simulink library "halout"  (R2021b)
settings: Solver=VariableStepAuto  StartTime=0.0  StopTime=10.0  RelTol=1e-3
undefined symbols (not defined in the file): C_TASK_5MS_S, FALSE, KHAL_CAN1FD1APS3E2E_flg, KHAL_CAN1FD1APS3TxReq_flg, KHAL_CAN1FD1VCU2E2E_flg, KHAL_CAN1FD1VCU2TxReq_flg, KHAL_CAN1FD1VCU3E2E_flg, KHAL_CAN1FD1VCU3TxReq_flg, KHAL_CAN1TxReq_flg, KHAL_CAN1VMCFCM1E2E_flg, KHAL_CAN1VMCFCM1TxReq_flg, KHAL_CAN2TxReq_flg, KHAL_CAN3FD3VCU1toNIDECTxReq_flg, KHAL_CAN3FD3VCU1TxReq_flg, KHAL_CAN3FD3VCU2E2E_flg, KHAL_CAN3FD3VCU2toNIDECE2E_flg, KHAL_CAN3FD3VCU2toNIDECTxReq_flg, KHAL_CAN3FD3VCU2TxReq_flg, KHAL_CAN3TxReq_flg, KHAL_CAN4FD4CE1000E2E_flg, KHAL_CAN4FD4CE1000TxReq_flg, KHAL_CAN4TxReq_flg, KHAL_CAN5TxReq_flg, KHAL_CAN6FD6APS3E2E_flg, KHAL_CAN6FD6APS3TxReq_flg, KHAL_CAN6FD6VCU2E2E_flg, KHAL_CAN6FD6VCU2TxReq_flg, KHAL_CAN6TxReq_flg, ONE_INT, TRUE, ZERO_INT
libraries: FVT_lib x500, simulink x235
(part 20 of 25)

== system halout/HAL_OUT/CAN3/FD3_VCU2_0x153/Byte_12 ==
  Fr_UdcMax : Inport
  Fr_UdcMin : Inport  Port=2
  BitwiseOR : simulink/Logic and Bit Operations/Bitwise Operator  logicop=OR  UseBitMask=off  NumInputPorts=2  BitMask=bin2dec('11011001')  BitMaskRealWorld=Stored Integer
  SignalPack : FVT_lib/hal/SignalPack  RightShiftCnt=0  BitMask=2^4-1  LeftShiftCnt=4
  SignalPack1 : FVT_lib/hal/SignalPack  RightShiftCnt=8  BitMask=2^4-1  LeftShiftCnt=0
  UnitConverter : DataTypeConversion  OutDataTypeStr=uint8  RndMeth=Round
  UnitConverter1 : DataTypeConversion  OutDataTypeStr=uint16  RndMeth=Round
  UnitConverter2 : DataTypeConversion  OutDataTypeStr=uint8  RndMeth=Round
  UnitConverter3 : DataTypeConversion  OutDataTypeStr=uint16  RndMeth=Round
  Byte_12 : Outport
  wires:
  BitwiseOR/1 -> Byte_12/1
  UnitConverter/1 -> BitwiseOR/1
  SignalPack/1 -> UnitConverter/1
  UnitConverter1/1 -> SignalPack/1
  Fr_UdcMax/1 -> UnitConverter1/1
  UnitConverter2/1 -> BitwiseOR/2
  SignalPack1/1 -> UnitConverter2/1
  UnitConverter3/1 -> SignalPack1/1
  Fr_UdcMin/1 -> UnitConverter3/1

== system halout/HAL_OUT/CAN3/FD3_VCU2_0x153/Byte_13 ==
  Fr_UdcMin : Inport
  BitwiseOR : simulink/Logic and Bit Operations/Bitwise Operator  logicop=OR  UseBitMask=off  BitMask=bin2dec('11011001')  BitMaskRealWorld=Stored Integer
  SignalPack : FVT_lib/hal/SignalPack  RightShiftCnt=0  BitMask=2^8-1  LeftShiftCnt=0
  UnitConverter : DataTypeConversion  OutDataTypeStr=uint8  RndMeth=Round
  UnitConverter1 : DataTypeConversion  OutDataTypeStr=uint16  RndMeth=Round
  Byte_13 : Outport
  wires:
  BitwiseOR/1 -> Byte_13/1
  UnitConverter/1 -> BitwiseOR/1
  SignalPack/1 -> UnitConverter/1
  UnitConverter1/1 -> SignalPack/1
  Fr_UdcMin/1 -> UnitConverter1/1

== system halout/HAL_OUT/CAN3/FD3_VCU2_0x153/Byte_14 ==
  Rr_TMTqReq : Inport
  BitwiseOR : simulink/Logic and Bit Operations/Bitwise Operator  logicop=OR  UseBitMask=off  BitMask=bin2dec('11011001')  BitMaskRealWorld=Stored Integer
  SignalPack : FVT_lib/hal/SignalPack  RightShiftCnt=8  BitMask=2^8-1  LeftShiftCnt=0
  UnitConverter : DataTypeConversion  OutDataTypeStr=uint8  RndMeth=Round
  UnitConverter1 : DataTypeConversion  OutDataTypeStr=uint16  RndMeth=Round
  convert_out : FVT_lib/hal/convert_out  gain=1  offset=-530
  Byte_14 : Outport
  wires:
  BitwiseOR/1 -> Byte_14/1
  UnitConverter/1 -> BitwiseOR/1
  SignalPack/1 -> UnitConverter/1
  UnitConverter1/1 -> SignalPack/1
  convert_out/1 -> UnitConverter1/1
  Rr_TMTqReq/1 -> convert_out/1

== system halout/HAL_OUT/CAN3/FD3_VCU2_0x153/Byte_15 ==
  Rr_TMTqReq : Inport
  BitwiseOR : simulink/Logic and Bit Operations/Bitwise Operator  logicop=OR  UseBitMask=off  BitMask=bin2dec('11011001')  BitMaskRealWorld=Stored Integer
  SignalPack : FVT_lib/hal/SignalPack  RightShiftCnt=0  BitMask=2^8-1  LeftShiftCnt=0
  UnitConverter : DataTypeConversion  OutDataTypeStr=uint8  RndMeth=Round
  UnitConverter1 : DataTypeConversion  OutDataTypeStr=uint16  RndMeth=Round
  convert_out : FVT_lib/hal/convert_out  gain=1  offset=-530
  Byte_15 : Outport
  wires:
  BitwiseOR/1 -> Byte_15/1
  UnitConverter/1 -> BitwiseOR/1
  SignalPack/1 -> UnitConverter/1
  UnitConverter1/1 -> SignalPack/1
  convert_out/1 -> UnitConverter1/1
  Rr_TMTqReq/1 -> convert_out/1

== system halout/HAL_OUT/CAN3/FD3_VCU2_0x153/Byte_16 ==
  Fr_TMTqReq : Inport
  BitwiseOR : simulink/Logic and Bit Operations/Bitwise Operator  logicop=OR  UseBitMask=off  BitMask=bin2dec('11011001')  BitMaskRealWorld=Stored Integer
  SignalPack : FVT_lib/hal/SignalPack  RightShiftCnt=8  BitMask=2^8-1  LeftShiftCnt=0
  UnitConverter : DataTypeConversion  OutDataTypeStr=uint8  RndMeth=Round
  UnitConverter1 : DataTypeConversion  OutDataTypeStr=uint16  RndMeth=Round
  convert_out : FVT_lib/hal/convert_out  gain=1  offset=-530
  Byte_16 : Outport
  wires:
  BitwiseOR/1 -> Byte_16/1
  UnitConverter/1 -> BitwiseOR/1
  SignalPack/1 -> UnitConverter/1
  UnitConverter1/1 -> SignalPack/1
  convert_out/1 -> UnitConverter1/1
  Fr_TMTqReq/1 -> convert_out/1

== system halout/HAL_OUT/CAN3/FD3_VCU2_0x153/Byte_17 ==
  Fr_TMTqReq : Inport
  BitwiseOR : simulink/Logic and Bit Operations/Bitwise Operator  logicop=OR  UseBitMask=off  BitMask=bin2dec('11011001')  BitMaskRealWorld=Stored Integer
  SignalPack : FVT_lib/hal/SignalPack  RightShiftCnt=0  BitMask=2^8-1  LeftShiftCnt=0
  UnitConverter : DataTypeConversion  OutDataTypeStr=uint8  RndMeth=Round
  UnitConverter1 : DataTypeConversion  OutDataTypeStr=uint16  RndMeth=Round
  convert_out : FVT_lib/hal/convert_out  gain=1  offset=-530
  Byte_17 : Outport
  wires:
  BitwiseOR/1 -> Byte_17/1
  UnitConverter/1 -> BitwiseOR/1
  SignalPack/1 -> UnitConverter/1
  UnitConverter1/1 -> SignalPack/1
  convert_out/1 -> UnitConverter1/1
  Fr_TMTqReq/1 -> convert_out/1

== system halout/HAL_OUT/CAN3/FD3_VCU2_0x153/Byte_18 ==
  Fr_IdcMax : Inport
  BitwiseOR : simulink/Logic and Bit Operations/Bitwise Operator  logicop=OR  UseBitMask=off  BitMask=bin2dec('11011001')  BitMaskRealWorld=Stored Integer
  SignalPack : FVT_lib/hal/SignalPack  RightShiftCnt=4  BitMask=2^8-1  LeftShiftCnt=0
  UnitConverter : DataTypeConversion  OutDataTypeStr=uint8  RndMeth=Round
  UnitConverter1 : DataTypeConversion  OutDataTypeStr=uint16  RndMeth=Round
  Byte_18 : Outport
  wires:
  BitwiseOR/1 -> Byte_18/1
  UnitConverter/1 -> BitwiseOR/1
  SignalPack/1 -> UnitConverter/1
  UnitConverter1/1 -> SignalPack/1
  Fr_IdcMax/1 -> UnitConverter1/1

== system halout/HAL_OUT/CAN3/FD3_VCU2_0x153/Byte_19 ==
  Fr_IdcMax : Inport
  Fr_IdcMin : Inport  Port=2
  BitwiseOR : simulink/Logic and Bit Operations/Bitwise Operator  logicop=OR  UseBitMask=off  NumInputPorts=2  BitMask=bin2dec('11011001')  BitMaskRealWorld=Stored Integer
  SignalPack : FVT_lib/hal/SignalPack  RightShiftCnt=0  BitMask=2^4-1  LeftShiftCnt=4
  SignalPack1 : FVT_lib/hal/SignalPack  RightShiftCnt=8  BitMask=2^4-1  LeftShiftCnt=0
  UnitConverter : DataTypeConversion  OutDataTypeStr=uint8  RndMeth=Round
  UnitConverter1 : DataTypeConversion  OutDataTypeStr=uint16  RndMeth=Round
  UnitConverter2 : DataTypeConversion  OutDataTypeStr=uint8  RndMeth=Round
  UnitConverter3 : DataTypeConversion  OutDataTypeStr=uint16  RndMeth=Round
  convert_out : FVT_lib/hal/convert_out  gain=1  offset=-1022
  Byte_19 : Outport
  wires:
  BitwiseOR/1 -> Byte_19/1
  UnitConverter/1 -> BitwiseOR/1
  SignalPack/1 -> UnitConverter/1
  UnitConverter1/1 -> SignalPack/1
  Fr_IdcMax/1 -> UnitConverter1/1
  UnitConverter2/1 -> BitwiseOR/2
  SignalPack1/1 -> UnitConverter2/1
  UnitConverter3/1 -> SignalPack1/1
  convert_out/1 -> UnitConverter3/1
  Fr_IdcMin/1 -> convert_out/1

== system halout/HAL_OUT/CAN3/FD3_VCU2_0x153/Byte_2 ==
  Rr_IdcMax : Inport
  BitwiseOR : simulink/Logic and Bit Operations/Bitwise Operator  logicop=OR  UseBitMask=off  BitMask=bin2dec('11011001')  BitMaskRealWorld=Stored Integer
  SignalPack : FVT_lib/hal/SignalPack  RightShiftCnt=4  BitMask=2^8-1  LeftShiftCnt=0
  UnitConverter : DataTypeConversion  OutDataTypeStr=uint8  RndMeth=Round
  UnitConverter1 : DataTypeConversion  OutDataTypeStr=uint16  RndMeth=Round
  Byte_2 : Outport
  wires:
  BitwiseOR/1 -> Byte_2/1
  UnitConverter/1 -> BitwiseOR/1
  SignalPack/1 -> UnitConverter/1
  UnitConverter1/1 -> SignalPack/1
  Rr_IdcMax/1 -> UnitConverter1/1

== system halout/HAL_OUT/CAN3/FD3_VCU2_0x153/Byte_20 ==
  Fr_IdcMin : Inport
  BitwiseOR : simulink/Logic and Bit Operations/Bitwise Operator  logicop=OR  UseBitMask=off  BitMask=bin2dec('11011001')  BitMaskRealWorld=Stored Integer
  SignalPack : FVT_lib/hal/SignalPack  RightShiftCnt=0  BitMask=2^8-1  LeftShiftCnt=0
  UnitConverter : DataTypeConversion  OutDataTypeStr=uint8  RndMeth=Round
  UnitConverter1 : DataTypeConversion  OutDataTypeStr=uint16  RndMeth=Round
  convert_out : FVT_lib/hal/convert_out  gain=1  offset=-1022
  Byte_20 : Outport
  wires:
  BitwiseOR/1 -> Byte_20/1
  UnitConverter/1 -> BitwiseOR/1
  SignalPack/1 -> UnitConverter/1
  UnitConverter1/1 -> SignalPack/1
  convert_out/1 -> UnitConverter1/1
  Fr_IdcMin/1 -> convert_out/1

== system halout/HAL_OUT/CAN3/FD3_VCU2_0x153/Byte_21 ==
  Fr_TorqMax : Inport
  BitwiseOR : simulink/Logic and Bit Operations/Bitwise Operator  logicop=OR  UseBitMask=off  BitMask=bin2dec('11011001')  BitMaskRealWorld=Stored Integer
  SignalPack : FVT_lib/hal/SignalPack  RightShiftCnt=4  BitMask=2^8-1  LeftShiftCnt=0
  UnitConverter : DataTypeConversion  OutDataTypeStr=uint8  RndMeth=Round
  UnitConverter1 : DataTypeConversion  OutDataTypeStr=uint16  RndMeth=Round
  Byte_21 : Outport
  wires:
  BitwiseOR/1 -> Byte_21/1
  UnitConverter/1 -> BitwiseOR/1
  SignalPack/1 -> UnitConverter/1
  UnitConverter1/1 -> SignalPack/1
  Fr_TorqMax/1 -> UnitConverter1/1

== system halout/HAL_OUT/CAN3/FD3_VCU2_0x153/Byte_22 ==
  Fr_TorqMax : Inport
  Fr_TorqMin : Inport  Port=2
  BitwiseOR : simulink/Logic and Bit Operations/Bitwise Operator  logicop=OR  UseBitMask=off  NumInputPorts=2  BitMask=bin2dec('11011001')  BitMaskRealWorld=Stored Integer
  SignalPack : FVT_lib/hal/SignalPack  RightShiftCnt=0  BitMask=2^4-1  LeftShiftCnt=4
  SignalPack1 : FVT_lib/hal/SignalPack  RightShiftCnt=8  BitMask=2^4-1  LeftShiftCnt=0
  UnitConverter : DataTypeConversion  OutDataTypeStr=uint8  RndMeth=Round
  UnitConverter1 : DataTypeConversion  OutDataTypeStr=uint16  RndMeth=Round
  UnitConverter2 : DataTypeConversion  OutDataTypeStr=uint8  RndMeth=Round
  UnitConverter3 : DataTypeConversion  OutDataTypeStr=uint16  RndMeth=Round
  convert_out : FVT_lib/hal/convert_out  gain=1  offset=-1022
  Byte_22 : Outport
  wires:
  BitwiseOR/1 -> Byte_22/1
  UnitConverter/1 -> BitwiseOR/1
  SignalPack/1 -> UnitConverter/1
  UnitConverter1/1 -> SignalPack/1
  Fr_TorqMax/1 -> UnitConverter1/1
  UnitConverter2/1 -> BitwiseOR/2
  SignalPack1/1 -> UnitConverter2/1
  UnitConverter3/1 -> SignalPack1/1
  convert_out/1 -> UnitConverter3/1
  Fr_TorqMin/1 -> convert_out/1

== system halout/HAL_OUT/CAN3/FD3_VCU2_0x153/Byte_23 ==
  Fr_TorqMin : Inport
  BitwiseOR : simulink/Logic and Bit Operations/Bitwise Operator  logicop=OR  UseBitMask=off  BitMask=bin2dec('11011001')  BitMaskRealWorld=Stored Integer
  SignalPack : FVT_lib/hal/SignalPack  RightShiftCnt=0  BitMask=2^8-1  LeftShiftCnt=0
  UnitConverter : DataTypeConversion  OutDataTypeStr=uint8  RndMeth=Round
  UnitConverter1 : DataTypeConversion  OutDataTypeStr=uint16  RndMeth=Round
  convert_out : FVT_lib/hal/convert_out  gain=1  offset=-1022
  Byte_23 : Outport
  wires:
  BitwiseOR/1 -> Byte_23/1
  UnitConverter/1 -> BitwiseOR/1
  SignalPack/1 -> UnitConverter/1
  UnitConverter1/1 -> SignalPack/1
  convert_out/1 -> UnitConverter1/1
  Fr_TorqMin/1 -> convert_out/1

== system halout/HAL_OUT/CAN3/FD3_VCU2_0x153/Byte_24 ==
  Fr_ActvDmpDisabReq : Inport
  Fr_MCUEnaReq : Inport  Port=2
  Rr_ActvDmpDisabReq : Inport  Port=3
  Rr_MCUEnaReq : Inport  Port=4
  BitwiseOR : simulink/Logic and Bit Operations/Bitwise Operator  logicop=OR  UseBitMask=off  NumInputPorts=4  BitMask=bin2dec('11011001')  BitMaskRealWorld=Stored Integer
  SignalPack : FVT_lib/hal/SignalPack  RightShiftCnt=0  BitMask=2^1-1  LeftShiftCnt=6
  SignalPack1 : FVT_lib/hal/SignalPack  RightShiftCnt=0  BitMask=2^1-1  LeftShiftCnt=7
  SignalPack2 : FVT_lib/hal/SignalPack  RightShiftCnt=0  BitMask=2^1-1  LeftShiftCnt=4
  SignalPack3 : FVT_lib/hal/SignalPack  RightShiftCnt=0  BitMask=2^1-1  LeftShiftCnt=5
  UnitConverter{,1..7} (8 alike) : DataTypeConversion  OutDataTypeStr=uint8  RndMeth=Round
  Byte_24 : Outport
  wires:
  BitwiseOR/1 -> Byte_24/1
  UnitConverter/1 -> BitwiseOR/1
  SignalPack/1 -> UnitConverter/1
  UnitConverter1/1 -> SignalPack/1
  Fr_ActvDmpDisabReq/1 -> UnitConverter1/1
  UnitConverter2/1 -> BitwiseOR/2
  SignalPack1/1 -> UnitConverter2/1
  UnitConverter3/1 -> SignalPack1/1
  Fr_MCUEnaReq/1 -> UnitConverter3/1
  UnitConverter4/1 -> BitwiseOR/3
  SignalPack2/1 -> UnitConverter4/1
  UnitConverter5/1 -> SignalPack2/1
  Rr_ActvDmpDisabReq/1 -> UnitConverter5/1
  UnitConverter6/1 -> BitwiseOR/4
  SignalPack3/1 -> UnitConverter6/1
  UnitConverter7/1 -> SignalPack3/1
  Rr_MCUEnaReq/1 -> UnitConverter7/1

== system halout/HAL_OUT/CAN3/FD3_VCU2_0x153/Byte_3 ==
  Rr_IdcMax : Inport
  Rr_IdcMin : Inport  Port=2
  BitwiseOR : simulink/Logic and Bit Operations/Bitwise Operator  logicop=OR  UseBitMask=off  NumInputPorts=2  BitMask=bin2dec('11011001')  BitMaskRealWorld=Stored Integer
  SignalPack : FVT_lib/hal/SignalPack  RightShiftCnt=0  BitMask=2^4-1  LeftShiftCnt=4
  SignalPack1 : FVT_lib/hal/SignalPack  RightShiftCnt=8  BitMask=2^4-1  LeftShiftCnt=0
  UnitConverter : DataTypeConversion  OutDataTypeStr=uint8  RndMeth=Round
  UnitConverter1 : DataTypeConversion  OutDataTypeStr=uint16  RndMeth=Round
  UnitConverter2 : DataTypeConversion  OutDataTypeStr=uint8  RndMeth=Round
  UnitConverter3 : DataTypeConversion  OutDataTypeStr=uint16  RndMeth=Round
  convert_out : FVT_lib/hal/convert_out  gain=1  offset=-1022
  Byte_3 : Outport
  wires:
  BitwiseOR/1 -> Byte_3/1
  UnitConverter/1 -> BitwiseOR/1
  SignalPack/1 -> UnitConverter/1
  UnitConverter1/1 -> SignalPack/1
  Rr_IdcMax/1 -> UnitConverter1/1
  UnitConverter2/1 -> BitwiseOR/2
  SignalPack1/1 -> UnitConverter2/1
  UnitConverter3/1 -> SignalPack1/1
  convert_out/1 -> UnitConverter3/1
  Rr_IdcMin/1 -> convert_out/1

== system halout/HAL_OUT/CAN3/FD3_VCU2_0x153/Byte_4 ==
  Rr_IdcMin : Inport
  BitwiseOR : simulink/Logic and Bit Operations/Bitwise Operator  logicop=OR  UseBitMask=off  BitMask=bin2dec('11011001')  BitMaskRealWorld=Stored Integer
  SignalPack : FVT_lib/hal/SignalPack  RightShiftCnt=0  BitMask=2^8-1  LeftShiftCnt=0
  UnitConverter : DataTypeConversion  OutDataTypeStr=uint8  RndMeth=Round
  UnitConverter1 : DataTypeConversion  OutDataTypeStr=uint16  RndMeth=Round
  convert_out : FVT_lib/hal/convert_out  gain=1  offset=-1022
  Byte_4 : Outport
  wires:
  BitwiseOR/1 -> Byte_4/1
  UnitConverter/1 -> BitwiseOR/1
  SignalPack/1 -> UnitConverter/1
  UnitConverter1/1 -> SignalPack/1
  convert_out/1 -> UnitConverter1/1
  Rr_IdcMin/1 -> convert_out/1

== system halout/HAL_OUT/CAN3/FD3_VCU2_0x153/Byte_5 ==
  Rr_TorqMax : Inport
  BitwiseOR : simulink/Logic and Bit Operations/Bitwise Operator  logicop=OR  UseBitMask=off  BitMask=bin2dec('11011001')  BitMaskRealWorld=Stored Integer
  SignalPack : FVT_lib/hal/SignalPack  RightShiftCnt=4  BitMask=2^8-1  LeftShiftCnt=0
  UnitConverter : DataTypeConversion  OutDataTypeStr=uint8  RndMeth=Round
  UnitConverter1 : DataTypeConversion  OutDataTypeStr=uint16  RndMeth=Round
  Byte_5 : Outport
  wires:
  BitwiseOR/1 -> Byte_5/1
  UnitConverter/1 -> BitwiseOR/1
  SignalPack/1 -> UnitConverter/1
  UnitConverter1/1 -> SignalPack/1
  Rr_TorqMax/1 -> UnitConverter1/1

== system halout/HAL_OUT/CAN3/FD3_VCU2_0x153/Byte_6 ==
  Rr_TorqMax : Inport
  Rr_TorqMin : Inport  Port=2
  BitwiseOR : simulink/Logic and Bit Operations/Bitwise Operator  logicop=OR  UseBitMask=off  NumInputPorts=2  BitMask=bin2dec('11011001')  BitMaskRealWorld=Stored Integer
  SignalPack : FVT_lib/hal/SignalPack  RightShiftCnt=0  BitMask=2^4-1  LeftShiftCnt=4
  SignalPack1 : FVT_lib/hal/SignalPack  RightShiftCnt=8  BitMask=2^4-1  LeftShiftCnt=0
  UnitConverter : DataTypeConversion  OutDataTypeStr=uint8  RndMeth=Round
  UnitConverter1 : DataTypeConversion  OutDataTypeStr=uint16  RndMeth=Round
  UnitConverter2 : DataTypeConversion  OutDataTypeStr=uint8  RndMeth=Round
  UnitConverter3 : DataTypeConversion  OutDataTypeStr=uint16  RndMeth=Round
  convert_out : FVT_lib/hal/convert_out  gain=1  offset=-1022
  Byte_6 : Outport
  wires:
  BitwiseOR/1 -> Byte_6/1
  UnitConverter/1 -> BitwiseOR/1
  SignalPack/1 -> UnitConverter/1
  UnitConverter1/1 -> SignalPack/1
  Rr_TorqMax/1 -> UnitConverter1/1
  UnitConverter2/1 -> BitwiseOR/2
  SignalPack1/1 -> UnitConverter2/1
  UnitConverter3/1 -> SignalPack1/1
  convert_out/1 -> UnitConverter3/1
  Rr_TorqMin/1 -> convert_out/1

== system halout/HAL_OUT/CAN3/FD3_VCU2_0x153/Byte_7 ==
  Rr_TorqMin : Inport
  BitwiseOR : simulink/Logic and Bit Operations/Bitwise Operator  logicop=OR  UseBitMask=off  BitMask=bin2dec('11011001')  BitMaskRealWorld=Stored Integer
  SignalPack : FVT_lib/hal/SignalPack  RightShiftCnt=0  BitMask=2^8-1  LeftShiftCnt=0
  UnitConverter : DataTypeConversion  OutDataTypeStr=uint8  RndMeth=Round
  UnitConverter1 : DataTypeConversion  OutDataTypeStr=uint16  RndMeth=Round
  convert_out : FVT_lib/hal/convert_out  gain=1  offset=-1022
  Byte_7 : Outport
  wires:
  BitwiseOR/1 -> Byte_7/1
  UnitConverter/1 -> BitwiseOR/1
  SignalPack/1 -> UnitConverter/1
  UnitConverter1/1 -> SignalPack/1
  convert_out/1 -> UnitConverter1/1
  Rr_TorqMin/1 -> convert_out/1

== system halout/HAL_OUT/CAN3/FD3_VCU2_0x153/Byte_8 ==
  Rr_UdcMax : Inport
  BitwiseOR : simulink/Logic and Bit Operations/Bitwise Operator  logicop=OR  UseBitMask=off  BitMask=bin2dec('11011001')  BitMaskRealWorld=Stored Integer
  SignalPack : FVT_lib/hal/SignalPack  RightShiftCnt=4  BitMask=2^8-1  LeftShiftCnt=0
  UnitConverter : DataTypeConversion  OutDataTypeStr=uint8  RndMeth=Round
  UnitConverter1 : DataTypeConversion  OutDataTypeStr=uint16  RndMeth=Round
  Byte_8 : Outport
  wires:
  BitwiseOR/1 -> Byte_8/1
  UnitConverter/1 -> BitwiseOR/1
  SignalPack/1 -> UnitConverter/1
  UnitConverter1/1 -> SignalPack/1
  Rr_UdcMax/1 -> UnitConverter1/1

== system halout/HAL_OUT/CAN3/FD3_VCU2_0x153/Byte_9 ==
  Rr_UdcMax : Inport
  Rr_UdcMin : Inport  Port=2
  BitwiseOR : simulink/Logic and Bit Operations/Bitwise Operator  logicop=OR  UseBitMask=off  NumInputPorts=2  BitMask=bin2dec('11011001')  BitMaskRealWorld=Stored Integer
  SignalPack : FVT_lib/hal/SignalPack  RightShiftCnt=0  BitMask=2^4-1  LeftShiftCnt=4
  SignalPack1 : FVT_lib/hal/SignalPack  RightShiftCnt=8  BitMask=2^4-1  LeftShiftCnt=0
  UnitConverter : DataTypeConversion  OutDataTypeStr=uint8  RndMeth=Round
  UnitConverter1 : DataTypeConversion  OutDataTypeStr=uint16  RndMeth=Round
  UnitConverter2 : DataTypeConversion  OutDataTypeStr=uint8  RndMeth=Round
  UnitConverter3 : DataTypeConversion  OutDataTypeStr=uint16  RndMeth=Round
  Byte_9 : Outport
  wires:
  BitwiseOR/1 -> Byte_9/1
  UnitConverter/1 -> BitwiseOR/1
  SignalPack/1 -> UnitConverter/1
  UnitConverter1/1 -> SignalPack/1
  Rr_UdcMax/1 -> UnitConverter1/1
  UnitConverter2/1 -> BitwiseOR/2
  SignalPack1/1 -> UnitConverter2/1
  UnitConverter3/1 -> SignalPack1/1
  Rr_UdcMin/1 -> UnitConverter3/1

== system halout/HAL_OUT/CAN3/FD3_VCU2_0x153/CRC8_IfAction_Tx ==
  CAN_E2E_flg : Inport
  DataID1 : Inport  Port=2
  DataID2 : Inport  Port=3
  RawData : Inport  Port=4
  Data Type Conversion : DataTypeConversion  OutDataTypeStr=uint8
  If : If
  If Action Subsystem : Subsystem  TreatAsAtomicUnit=on
  If Action Subsystem1 : Subsystem  TreatAsAtomicUnit=on
  Merge : Merge
  CRC8 : Outport
  wires:
  If/2 -> If Action Subsystem/Action
  If/1 -> If Action Subsystem1/Action
  CAN_E2E_flg/1 -> [CAN_E2E_flg]
  DataID1/1 -> [DataID1]
  DataID2/1 -> [DataID2]
  RawData/1 -> [RawData]
  [CAN_E2E_flg] -> Data Type Conversion/1
  [DataID1] -> If Action Subsystem1/1(CAN_E2E_ID1)
  [DataID2] -> If Action Subsystem1/2(CAN_E2E_ID2)
  [RawData] -> If Action Subsystem1/3(Byte1)
  [RawData] -> If Action Subsystem/1(Byte1)
  If Action Subsystem1/1(CRC8_E2EResult) -> Merge/1
  If Action Subsystem/1(CRC8_Result) -> Merge/2
  Merge/1 -> CRC8/1
  Data Type Conversion/1 -> If/1

== system halout/HAL_OUT/CAN3/FD3_VCU2_0x153/CSVCU2CAN1 ==
  CSVCU2CAN1 : Inport
  Data Type Conversion : DataTypeConversion  OutDataTypeStr=uint8  RndMeth=Round
  CAN3_CS_VCU2_CAN1 : Outport
  wires:
  Data Type Conversion/1 -> CAN3_CS_VCU2_CAN1/1
  CSVCU2CAN1/1 -> Data Type Conversion/1

== system halout/HAL_OUT/CAN3/FD3_VCU2_0x153/FrActvDmpDisabReq ==
  FrActvDmpDisabReq : Inport
  Data Type Conversion : DataTypeConversion  OutDataTypeStr=uint8  RndMeth=Round
  CAN3_Fr_ActvDmpDisabReq : Outport
  wires:
  Data Type Conversion/1 -> CAN3_Fr_ActvDmpDisabReq/1
  FrActvDmpDisabReq/1 -> Data Type Conversion/1

== system halout/HAL_OUT/CAN3/FD3_VCU2_0x153/FrIdcMax ==
  FrIdcMax : Inport
  Data Type Conversion : DataTypeConversion  OutDataTypeStr=uint16  RndMeth=Round
  CAN3_Fr_IdcMax : Outport
  wires:
  Data Type Conversion/1 -> CAN3_Fr_IdcMax/1
  FrIdcMax/1 -> Data Type Conversion/1

== system halout/HAL_OUT/CAN3/FD3_VCU2_0x153/FrIdcMin ==
  FrIdcMin : Inport
  Data Type Conversion : DataTypeConversion  OutDataTypeStr=uint16  RndMeth=Round
  convert_out : FVT_lib/hal/convert_out  gain=1  offset=-1022
  CAN3_Fr_IdcMin : Outport
  wires:
  Data Type Conversion/1 -> CAN3_Fr_IdcMin/1
  convert_out/1 -> Data Type Conversion/1
  FrIdcMin/1 -> convert_out/1

== system halout/HAL_OUT/CAN3/FD3_VCU2_0x153/FrMCUEnaReq ==
  FrMCUEnaReq : Inport
  Data Type Conversion : DataTypeConversion  OutDataTypeStr=uint8  RndMeth=Round
  CAN3_Fr_MCUEnaReq : Outport
  wires:
  Data Type Conversion/1 -> CAN3_Fr_MCUEnaReq/1
  FrMCUEnaReq/1 -> Data Type Conversion/1

== system halout/HAL_OUT/CAN3/FD3_VCU2_0x153/FrTMTqReq ==
  FrTMTqReq : Inport
  Data Type Conversion : DataTypeConversion  OutDataTypeStr=uint16  RndMeth=Round
  convert_out : FVT_lib/hal/convert_out  gain=1  offset=-530
  CAN3_Fr_TMTqReq : Outport
  wires:
  Data Type Conversion/1 -> CAN3_Fr_TMTqReq/1
  convert_out/1 -> Data Type Conversion/1
  FrTMTqReq/1 -> convert_out/1

== system halout/HAL_OUT/CAN3/FD3_VCU2_0x153/FrTorqMax ==
  FrTorqMax : Inport
  Data Type Conversion : DataTypeConversion  OutDataTypeStr=uint16  RndMeth=Round
  CAN3_Fr_TorqMax : Outport
  wires:
  Data Type Conversion/1 -> CAN3_Fr_TorqMax/1
  FrTorqMax/1 -> Data Type Conversion/1

== system halout/HAL_OUT/CAN3/FD3_VCU2_0x153/FrTorqMin ==
  FrTorqMin : Inport
  Data Type Conversion : DataTypeConversion  OutDataTypeStr=uint16  RndMeth=Round
  convert_out : FVT_lib/hal/convert_out  gain=1  offset=-1022
  CAN3_Fr_TorqMin : Outport
  wires:
  Data Type Conversion/1 -> CAN3_Fr_TorqMin/1
  convert_out/1 -> Data Type Conversion/1
  FrTorqMin/1 -> convert_out/1

== system halout/HAL_OUT/CAN3/FD3_VCU2_0x153/FrUdcMax ==
  FrUdcMax : Inport
  Data Type Conversion : DataTypeConversion  OutDataTypeStr=uint16  RndMeth=Round
  CAN3_Fr_UdcMax : Outport
  wires:
  Data Type Conversion/1 -> CAN3_Fr_UdcMax/1
  FrUdcMax/1 -> Data Type Conversion/1

== system halout/HAL_OUT/CAN3/FD3_VCU2_0x153/FrUdcMin ==
  FrUdcMin : Inport
  Data Type Conversion : DataTypeConversion  OutDataTypeStr=uint16  RndMeth=Round
  CAN3_Fr_UdcMin : Outport
  wires:
  Data Type Conversion/1 -> CAN3_Fr_UdcMin/1
  FrUdcMin/1 -> Data Type Conversion/1

== system halout/HAL_OUT/CAN3/FD3_VCU2_0x153/RCVCU2CAN1 ==
  RCVCU2CAN1 : Inport
  Data Type Conversion : DataTypeConversion  OutDataTypeStr=uint8  RndMeth=Round
  CAN3_RC_VCU2_CAN1 : Outport
  wires:
  Data Type Conversion/1 -> CAN3_RC_VCU2_CAN1/1
  RCVCU2CAN1/1 -> Data Type Conversion/1

== system halout/HAL_OUT/CAN3/FD3_VCU2_0x153/RrActvDmpDisabReq ==
  RrActvDmpDisabReq : Inport
  Data Type Conversion : DataTypeConversion  OutDataTypeStr=uint8  RndMeth=Round
  CAN3_Rr_ActvDmpDisabReq : Outport
  wires:
  Data Type Conversion/1 -> CAN3_Rr_ActvDmpDisabReq/1
  RrActvDmpDisabReq/1 -> Data Type Conversion/1

== system halout/HAL_OUT/CAN3/FD3_VCU2_0x153/RrIdcMax ==
  RrIdcMax : Inport
  Data Type Conversion : DataTypeConversion  OutDataTypeStr=uint16  RndMeth=Round
  CAN3_Rr_IdcMax : Outport
  wires:
  Data Type Conversion/1 -> CAN3_Rr_IdcMax/1
  RrIdcMax/1 -> Data Type Conversion/1

== system halout/HAL_OUT/CAN3/FD3_VCU2_0x153/RrIdcMin ==
  RrIdcMin : Inport
  Data Type Conversion : DataTypeConversion  OutDataTypeStr=uint16  RndMeth=Round
  convert_out : FVT_lib/hal/convert_out  gain=1  offset=-1022
  CAN3_Rr_IdcMin : Outport
  wires:
  Data Type Conversion/1 -> CAN3_Rr_IdcMin/1
  convert_out/1 -> Data Type Conversion/1
  RrIdcMin/1 -> convert_out/1

== system halout/HAL_OUT/CAN3/FD3_VCU2_0x153/RrMCUEnaReq ==
  RrMCUEnaReq : Inport
  Data Type Conversion : DataTypeConversion  OutDataTypeStr=uint8  RndMeth=Round
  CAN3_Rr_MCUEnaReq : Outport
  wires:
  Data Type Conversion/1 -> CAN3_Rr_MCUEnaReq/1
  RrMCUEnaReq/1 -> Data Type Conversion/1

== system halout/HAL_OUT/CAN3/FD3_VCU2_0x153/RrTMTqReq ==
  RrTMTqReq : Inport
  Data Type Conversion : DataTypeConversion  OutDataTypeStr=uint16  RndMeth=Round
  convert_out : FVT_lib/hal/convert_out  gain=1  offset=-530
  CAN3_Rr_TMTqReq : Outport
  wires:
  Data Type Conversion/1 -> CAN3_Rr_TMTqReq/1
  convert_out/1 -> Data Type Conversion/1
  RrTMTqReq/1 -> convert_out/1

== system halout/HAL_OUT/CAN3/FD3_VCU2_0x153/RrTorqMax ==
  RrTorqMax : Inport
  Data Type Conversion : DataTypeConversion  OutDataTypeStr=uint16  RndMeth=Round
  CAN3_Rr_TorqMax : Outport
  wires:
  Data Type Conversion/1 -> CAN3_Rr_TorqMax/1
  RrTorqMax/1 -> Data Type Conversion/1

== system halout/HAL_OUT/CAN3/FD3_VCU2_0x153/RrTorqMin ==
  RrTorqMin : Inport
  Data Type Conversion : DataTypeConversion  OutDataTypeStr=uint16  RndMeth=Round
  convert_out : FVT_lib/hal/convert_out  gain=1  offset=-1022
  CAN3_Rr_TorqMin : Outport
  wires:
  Data Type Conversion/1 -> CAN3_Rr_TorqMin/1
  convert_out/1 -> Data Type Conversion/1
  RrTorqMin/1 -> convert_out/1

== system halout/HAL_OUT/CAN3/FD3_VCU2_0x153/RrUdcMax ==
  RrUdcMax : Inport
  Data Type Conversion : DataTypeConversion  OutDataTypeStr=uint16  RndMeth=Round
  CAN3_Rr_UdcMax : Outport
  wires:
  Data Type Conversion/1 -> CAN3_Rr_UdcMax/1
  RrUdcMax/1 -> Data Type Conversion/1

== system halout/HAL_OUT/CAN3/FD3_VCU2_0x153/RrUdcMin ==
  RrUdcMin : Inport
  Data Type Conversion : DataTypeConversion  OutDataTypeStr=uint16  RndMeth=Round
  CAN3_Rr_UdcMin : Outport
  wires:
  Data Type Conversion/1 -> CAN3_Rr_UdcMin/1
  RrUdcMin/1 -> Data Type Conversion/1

== system halout/HAL_OUT/CAN3/FD3_VCU2_toNIDEC_0x154/Byte_0 ==
  CS_VCU2_CAN1_toNidec : Inport
  BitwiseOR : simulink/Logic and Bit Operations/Bitwise Operator  logicop=OR  UseBitMask=off  BitMask=bin2dec('11011001')  BitMaskRealWorld=Stored Integer
  SignalPack : FVT_lib/hal/SignalPack  RightShiftCnt=0  BitMask=2^8-1  LeftShiftCnt=0
  UnitConverter : DataTypeConversion  OutDataTypeStr=uint8  RndMeth=Round
  UnitConverter1 : DataTypeConversion  OutDataTypeStr=uint8  RndMeth=Round
  Byte_0 : Outport
  wires:
  BitwiseOR/1 -> Byte_0/1
  UnitConverter/1 -> BitwiseOR/1
  SignalPack/1 -> UnitConverter/1
  UnitConverter1/1 -> SignalPack/1
  CS_VCU2_CAN1_toNidec/1 -> UnitConverter1/1

== system halout/HAL_OUT/CAN3/FD3_VCU2_toNIDEC_0x154/Byte_1 ==
  RC_VCU2_CAN1_toNidec : Inport
  BitwiseOR : simulink/Logic and Bit Operations/Bitwise Operator  logicop=OR  UseBitMask=off  BitMask=bin2dec('11011001')  BitMaskRealWorld=Stored Integer
  SignalPack : FVT_lib/hal/SignalPack  RightShiftCnt=0  BitMask=2^4-1  LeftShiftCnt=4
  UnitConverter : DataTypeConversion  OutDataTypeStr=uint8  RndMeth=Round
  UnitConverter1 : DataTypeConversion  OutDataTypeStr=uint8  RndMeth=Round
  Byte_1 : Outport
  wires:
  BitwiseOR/1 -> Byte_1/1
  UnitConverter/1 -> BitwiseOR/1
  SignalPack/1 -> UnitConverter/1
  UnitConverter1/1 -> SignalPack/1
  RC_VCU2_CAN1_toNidec/1 -> UnitConverter1/1

== system halout/HAL_OUT/CAN3/FD3_VCU2_toNIDEC_0x154/Byte_10 ==
  Rr_UdcMin_toNidec : Inport
  BitwiseOR : simulink/Logic and Bit Operations/Bitwise Operator  logicop=OR  UseBitMask=off  BitMask=bin2dec('11011001')  BitMaskRealWorld=Stored Integer
  SignalPack : FVT_lib/hal/SignalPack  RightShiftCnt=0  BitMask=2^8-1  LeftShiftCnt=0
  UnitConverter : DataTypeConversion  OutDataTypeStr=uint8  RndMeth=Round
  UnitConverter1 : DataTypeConversion  OutDataTypeStr=uint16  RndMeth=Round
  Byte_10 : Outport
  wires:
  BitwiseOR/1 -> Byte_10/1
  UnitConverter/1 -> BitwiseOR/1
  SignalPack/1 -> UnitConverter/1
  UnitConverter1/1 -> SignalPack/1
  Rr_UdcMin_toNidec/1 -> UnitConverter1/1

== system halout/HAL_OUT/CAN3/FD3_VCU2_toNIDEC_0x154/Byte_11 ==
  Fr_UdcMax_toNidec : Inport
  BitwiseOR : simulink/Logic and Bit Operations/Bitwise Operator  logicop=OR  UseBitMask=off  BitMask=bin2dec('11011001')  BitMaskRealWorld=Stored Integer
  SignalPack : FVT_lib/hal/SignalPack  RightShiftCnt=4  BitMask=2^8-1  LeftShiftCnt=0
  UnitConverter : DataTypeConversion  OutDataTypeStr=uint8  RndMeth=Round
  UnitConverter1 : DataTypeConversion  OutDataTypeStr=uint16  RndMeth=Round
  Byte_11 : Outport
  wires:
  BitwiseOR/1 -> Byte_11/1
  UnitConverter/1 -> BitwiseOR/1
  SignalPack/1 -> UnitConverter/1
  UnitConverter1/1 -> SignalPack/1
  Fr_UdcMax_toNidec/1 -> UnitConverter1/1

== system halout/HAL_OUT/CAN3/FD3_VCU2_toNIDEC_0x154/Byte_12 ==
  Fr_UdcMax_toNidec : Inport
  Fr_UdcMin_toNidec : Inport  Port=2
  BitwiseOR : simulink/Logic and Bit Operations/Bitwise Operator  logicop=OR  UseBitMask=off  NumInputPorts=2  BitMask=bin2dec('11011001')  BitMaskRealWorld=Stored Integer
  SignalPack : FVT_lib/hal/SignalPack  RightShiftCnt=0  BitMask=2^4-1  LeftShiftCnt=4
  SignalPack1 : FVT_lib/hal/SignalPack  RightShiftCnt=8  BitMask=2^4-1  LeftShiftCnt=0
  UnitConverter : DataTypeConversion  OutDataTypeStr=uint8  RndMeth=Round
  UnitConverter1 : DataTypeConversion  OutDataTypeStr=uint16  RndMeth=Round
  UnitConverter2 : DataTypeConversion  OutDataTypeStr=uint8  RndMeth=Round
  UnitConverter3 : DataTypeConversion  OutDataTypeStr=uint16  RndMeth=Round
  Byte_12 : Outport
  wires:
  BitwiseOR/1 -> Byte_12/1
  UnitConverter/1 -> BitwiseOR/1
  SignalPack/1 -> UnitConverter/1
  UnitConverter1/1 -> SignalPack/1
  Fr_UdcMax_toNidec/1 -> UnitConverter1/1
  UnitConverter2/1 -> BitwiseOR/2
  SignalPack1/1 -> UnitConverter2/1
  UnitConverter3/1 -> SignalPack1/1
  Fr_UdcMin_toNidec/1 -> UnitConverter3/1

== system halout/HAL_OUT/CAN3/FD3_VCU2_toNIDEC_0x154/Byte_13 ==
  Fr_UdcMin_toNidec : Inport
  BitwiseOR : simulink/Logic and Bit Operations/Bitwise Operator  logicop=OR  UseBitMask=off  BitMask=bin2dec('11011001')  BitMaskRealWorld=Stored Integer
  SignalPack : FVT_lib/hal/SignalPack  RightShiftCnt=0  BitMask=2^8-1  LeftShiftCnt=0
  UnitConverter : DataTypeConversion  OutDataTypeStr=uint8  RndMeth=Round
  UnitConverter1 : DataTypeConversion  OutDataTypeStr=uint16  RndMeth=Round
  Byte_13 : Outport
  wires:
  BitwiseOR/1 -> Byte_13/1
  UnitConverter/1 -> BitwiseOR/1
  SignalPack/1 -> UnitConverter/1
  UnitConverter1/1 -> SignalPack/1
  Fr_UdcMin_toNidec/1 -> UnitConverter1/1

== system halout/HAL_OUT/CAN3/FD3_VCU2_toNIDEC_0x154/Byte_14 ==
  Rr_TMTqReq_toNidec : Inport
  BitwiseOR : simulink/Logic and Bit Operations/Bitwise Operator  logicop=OR  UseBitMask=off  BitMask=bin2dec('11011001')  BitMaskRealWorld=Stored Integer
  SignalPack : FVT_lib/hal/SignalPack  RightShiftCnt=8  BitMask=2^8-1  LeftShiftCnt=0
  UnitConverter : DataTypeConversion  OutDataTypeStr=uint8  RndMeth=Round
  UnitConverter1 : DataTypeConversion  OutDataTypeStr=uint16  RndMeth=Round
  convert_out : FVT_lib/hal/convert_out  gain=1  offset=-530
  Byte_14 : Outport
  wires:
  BitwiseOR/1 -> Byte_14/1
  UnitConverter/1 -> BitwiseOR/1
  SignalPack/1 -> UnitConverter/1
  UnitConverter1/1 -> SignalPack/1
  convert_out/1 -> UnitConverter1/1
  Rr_TMTqReq_toNidec/1 -> convert_out/1

== system halout/HAL_OUT/CAN3/FD3_VCU2_toNIDEC_0x154/Byte_15 ==
  Rr_TMTqReq_toNidec : Inport
  BitwiseOR : simulink/Logic and Bit Operations/Bitwise Operator  logicop=OR  UseBitMask=off  BitMask=bin2dec('11011001')  BitMaskRealWorld=Stored Integer
  SignalPack : FVT_lib/hal/SignalPack  RightShiftCnt=0  BitMask=2^8-1  LeftShiftCnt=0
  UnitConverter : DataTypeConversion  OutDataTypeStr=uint8  RndMeth=Round
  UnitConverter1 : DataTypeConversion  OutDataTypeStr=uint16  RndMeth=Round
  convert_out : FVT_lib/hal/convert_out  gain=1  offset=-530
  Byte_15 : Outport
  wires:
  BitwiseOR/1 -> Byte_15/1
  UnitConverter/1 -> BitwiseOR/1
  SignalPack/1 -> UnitConverter/1
  UnitConverter1/1 -> SignalPack/1
  convert_out/1 -> UnitConverter1/1
  Rr_TMTqReq_toNidec/1 -> convert_out/1

== system halout/HAL_OUT/CAN3/FD3_VCU2_toNIDEC_0x154/Byte_16 ==
  Fr_TMTqReq_toNidec : Inport
  BitwiseOR : simulink/Logic and Bit Operations/Bitwise Operator  logicop=OR  UseBitMask=off  BitMask=bin2dec('11011001')  BitMaskRealWorld=Stored Integer
  SignalPack : FVT_lib/hal/SignalPack  RightShiftCnt=8  BitMask=2^8-1  LeftShiftCnt=0
  UnitConverter : DataTypeConversion  OutDataTypeStr=uint8  RndMeth=Round
  UnitConverter1 : DataTypeConversion  OutDataTypeStr=uint16  RndMeth=Round
  convert_out : FVT_lib/hal/convert_out  gain=1  offset=-530
  Byte_16 : Outport
  wires:
  BitwiseOR/1 -> Byte_16/1
  UnitConverter/1 -> BitwiseOR/1
  SignalPack/1 -> UnitConverter/1
  UnitConverter1/1 -> SignalPack/1
  convert_out/1 -> UnitConverter1/1
  Fr_TMTqReq_toNidec/1 -> convert_out/1

== system halout/HAL_OUT/CAN3/FD3_VCU2_toNIDEC_0x154/Byte_17 ==
  Fr_TMTqReq_toNidec : Inport
  BitwiseOR : simulink/Logic and Bit Operations/Bitwise Operator  logicop=OR  UseBitMask=off  BitMask=bin2dec('11011001')  BitMaskRealWorld=Stored Integer
  SignalPack : FVT_lib/hal/SignalPack  RightShiftCnt=0  BitMask=2^8-1  LeftShiftCnt=0
  UnitConverter : DataTypeConversion  OutDataTypeStr=uint8  RndMeth=Round
  UnitConverter1 : DataTypeConversion  OutDataTypeStr=uint16  RndMeth=Round
  convert_out : FVT_lib/hal/convert_out  gain=1  offset=-530
  Byte_17 : Outport
  wires:
  BitwiseOR/1 -> Byte_17/1
  UnitConverter/1 -> BitwiseOR/1
  SignalPack/1 -> UnitConverter/1
  UnitConverter1/1 -> SignalPack/1
  convert_out/1 -> UnitConverter1/1
  Fr_TMTqReq_toNidec/1 -> convert_out/1

== system halout/HAL_OUT/CAN3/FD3_VCU2_toNIDEC_0x154/Byte_18 ==
  Fr_IdcMax_toNidec : Inport
  BitwiseOR : simulink/Logic and Bit Operations/Bitwise Operator  logicop=OR  UseBitMask=off  BitMask=bin2dec('11011001')  BitMaskRealWorld=Stored Integer
  SignalPack : FVT_lib/hal/SignalPack  RightShiftCnt=4  BitMask=2^8-1  LeftShiftCnt=0
  UnitConverter : DataTypeConversion  OutDataTypeStr=uint8  RndMeth=Round
  UnitConverter1 : DataTypeConversion  OutDataTypeStr=uint16  RndMeth=Round
  Byte_18 : Outport
  wires:
  BitwiseOR/1 -> Byte_18/1
  UnitConverter/1 -> BitwiseOR/1
  SignalPack/1 -> UnitConverter/1
  UnitConverter1/1 -> SignalPack/1
  Fr_IdcMax_toNidec/1 -> UnitConverter1/1

== system halout/HAL_OUT/CAN3/FD3_VCU2_toNIDEC_0x154/Byte_19 ==
  Fr_IdcMax_toNidec : Inport
  Fr_IdcMin_toNidec : Inport  Port=2
  BitwiseOR : simulink/Logic and Bit Operations/Bitwise Operator  logicop=OR  UseBitMask=off  NumInputPorts=2  BitMask=bin2dec('11011001')  BitMaskRealWorld=Stored Integer
  SignalPack : FVT_lib/hal/SignalPack  RightShiftCnt=0  BitMask=2^4-1  LeftShiftCnt=4
  SignalPack1 : FVT_lib/hal/SignalPack  RightShiftCnt=8  BitMask=2^4-1  LeftShiftCnt=0
  UnitConverter : DataTypeConversion  OutDataTypeStr=uint8  RndMeth=Round
  UnitConverter1 : DataTypeConversion  OutDataTypeStr=uint16  RndMeth=Round
  UnitConverter2 : DataTypeConversion  OutDataTypeStr=uint8  RndMeth=Round
  UnitConverter3 : DataTypeConversion  OutDataTypeStr=uint16  RndMeth=Round
  convert_out : FVT_lib/hal/convert_out  gain=1  offset=-1022
  Byte_19 : Outport
  wires:
  BitwiseOR/1 -> Byte_19/1
  UnitConverter/1 -> BitwiseOR/1
  SignalPack/1 -> UnitConverter/1
  UnitConverter1/1 -> SignalPack/1
  Fr_IdcMax_toNidec/1 -> UnitConverter1/1
  UnitConverter2/1 -> BitwiseOR/2
  SignalPack1/1 -> UnitConverter2/1
  UnitConverter3/1 -> SignalPack1/1
  convert_out/1 -> UnitConverter3/1
  Fr_IdcMin_toNidec/1 -> convert_out/1

== system halout/HAL_OUT/CAN3/FD3_VCU2_toNIDEC_0x154/Byte_2 ==
  Rr_IdcMax_toNidec : Inport
  BitwiseOR : simulink/Logic and Bit Operations/Bitwise Operator  logicop=OR  UseBitMask=off  BitMask=bin2dec('11011001')  BitMaskRealWorld=Stored Integer
  SignalPack : FVT_lib/hal/SignalPack  RightShiftCnt=4  BitMask=2^8-1  LeftShiftCnt=0
  UnitConverter : DataTypeConversion  OutDataTypeStr=uint8  RndMeth=Round
  UnitConverter1 : DataTypeConversion  OutDataTypeStr=uint16  RndMeth=Round
  Byte_2 : Outport
  wires:
  BitwiseOR/1 -> Byte_2/1
  UnitConverter/1 -> BitwiseOR/1
  SignalPack/1 -> UnitConverter/1
  UnitConverter1/1 -> SignalPack/1
  Rr_IdcMax_toNidec/1 -> UnitConverter1/1

== system halout/HAL_OUT/CAN3/FD3_VCU2_toNIDEC_0x154/Byte_20 ==
  Fr_IdcMin_toNidec : Inport
  BitwiseOR : simulink/Logic and Bit Operations/Bitwise Operator  logicop=OR  UseBitMask=off  BitMask=bin2dec('11011001')  BitMaskRealWorld=Stored Integer
  SignalPack : FVT_lib/hal/SignalPack  RightShiftCnt=0  BitMask=2^8-1  LeftShiftCnt=0
  UnitConverter : DataTypeConversion  OutDataTypeStr=uint8  RndMeth=Round
  UnitConverter1 : DataTypeConversion  OutDataTypeStr=uint16  RndMeth=Round
  convert_out : FVT_lib/hal/convert_out  gain=1  offset=-1022
  Byte_20 : Outport
  wires:
  BitwiseOR/1 -> Byte_20/1
  UnitConverter/1 -> BitwiseOR/1
  SignalPack/1 -> UnitConverter/1
  UnitConverter1/1 -> SignalPack/1
  convert_out/1 -> UnitConverter1/1
  Fr_IdcMin_toNidec/1 -> convert_out/1

== system halout/HAL_OUT/CAN3/FD3_VCU2_toNIDEC_0x154/Byte_21 ==
  Fr_TorqMax_toNidec : Inport
  BitwiseOR : simulink/Logic and Bit Operations/Bitwise Operator  logicop=OR  UseBitMask=off  BitMask=bin2dec('11011001')  BitMaskRealWorld=Stored Integer
  SignalPack : FVT_lib/hal/SignalPack  RightShiftCnt=4  BitMask=2^8-1  LeftShiftCnt=0
  UnitConverter : DataTypeConversion  OutDataTypeStr=uint8  RndMeth=Round
  UnitConverter1 : DataTypeConversion  OutDataTypeStr=uint16  RndMeth=Round
  Byte_21 : Outport
  wires:
  BitwiseOR/1 -> Byte_21/1
  UnitConverter/1 -> BitwiseOR/1
  SignalPack/1 -> UnitConverter/1
  UnitConverter1/1 -> SignalPack/1
  Fr_TorqMax_toNidec/1 -> UnitConverter1/1

== system halout/HAL_OUT/CAN3/FD3_VCU2_toNIDEC_0x154/Byte_22 ==
  Fr_TorqMax_toNidec : Inport
  Fr_TorqMin_toNidec : Inport  Port=2
  BitwiseOR : simulink/Logic and Bit Operations/Bitwise Operator  logicop=OR  UseBitMask=off  NumInputPorts=2  BitMask=bin2dec('11011001')  BitMaskRealWorld=Stored Integer
  SignalPack : FVT_lib/hal/SignalPack  RightShiftCnt=0  BitMask=2^4-1  LeftShiftCnt=4
  SignalPack1 : FVT_lib/hal/SignalPack  RightShiftCnt=8  BitMask=2^4-1  LeftShiftCnt=0
  UnitConverter : DataTypeConversion  OutDataTypeStr=uint8  RndMeth=Round
  UnitConverter1 : DataTypeConversion  OutDataTypeStr=uint16  RndMeth=Round
  UnitConverter2 : DataTypeConversion  OutDataTypeStr=uint8  RndMeth=Round
  UnitConverter3 : DataTypeConversion  OutDataTypeStr=uint16  RndMeth=Round
  convert_out : FVT_lib/hal/convert_out  gain=1  offset=-1022
  Byte_22 : Outport
  wires:
  BitwiseOR/1 -> Byte_22/1
  UnitConverter/1 -> BitwiseOR/1
  SignalPack/1 -> UnitConverter/1
  UnitConverter1/1 -> SignalPack/1
  Fr_TorqMax_toNidec/1 -> UnitConverter1/1
  UnitConverter2/1 -> BitwiseOR/2
  SignalPack1/1 -> UnitConverter2/1
  UnitConverter3/1 -> SignalPack1/1
  convert_out/1 -> UnitConverter3/1
  Fr_TorqMin_toNidec/1 -> convert_out/1

== system halout/HAL_OUT/CAN3/FD3_VCU2_toNIDEC_0x154/Byte_23 ==
  Fr_TorqMin_toNidec : Inport
  BitwiseOR : simulink/Logic and Bit Operations/Bitwise Operator  logicop=OR  UseBitMask=off  BitMask=bin2dec('11011001')  BitMaskRealWorld=Stored Integer
  SignalPack : FVT_lib/hal/SignalPack  RightShiftCnt=0  BitMask=2^8-1  LeftShiftCnt=0
  UnitConverter : DataTypeConversion  OutDataTypeStr=uint8  RndMeth=Round
  UnitConverter1 : DataTypeConversion  OutDataTypeStr=uint16  RndMeth=Round
  convert_out : FVT_lib/hal/convert_out  gain=1  offset=-1022
  Byte_23 : Outport
  wires:
  BitwiseOR/1 -> Byte_23/1
  UnitConverter/1 -> BitwiseOR/1
  SignalPack/1 -> UnitConverter/1
  UnitConverter1/1 -> SignalPack/1
  convert_out/1 -> UnitConverter1/1
  Fr_TorqMin_toNidec/1 -> convert_out/1

== system halout/HAL_OUT/CAN3/FD3_VCU2_toNIDEC_0x154/Byte_3 ==
  Rr_IdcMax_toNidec : Inport
  Rr_IdcMin_toNidec : Inport  Port=2
  BitwiseOR : simulink/Logic and Bit Operations/Bitwise Operator  logicop=OR  UseBitMask=off  NumInputPorts=2  BitMask=bin2dec('11011001')  BitMaskRealWorld=Stored Integer
  SignalPack : FVT_lib/hal/SignalPack  RightShiftCnt=0  BitMask=2^4-1  LeftShiftCnt=4
  SignalPack1 : FVT_lib/hal/SignalPack  RightShiftCnt=8  BitMask=2^4-1  LeftShiftCnt=0
  UnitConverter : DataTypeConversion  OutDataTypeStr=uint8  RndMeth=Round
  UnitConverter1 : DataTypeConversion  OutDataTypeStr=uint16  RndMeth=Round
  UnitConverter2 : DataTypeConversion  OutDataTypeStr=uint8  RndMeth=Round
  UnitConverter3 : DataTypeConversion  OutDataTypeStr=uint16  RndMeth=Round
  convert_out : FVT_lib/hal/convert_out  gain=1  offset=-1022
  Byte_3 : Outport
  wires:
  BitwiseOR/1 -> Byte_3/1
  UnitConverter/1 -> BitwiseOR/1
  SignalPack/1 -> UnitConverter/1
  UnitConverter1/1 -> SignalPack/1
  Rr_IdcMax_toNidec/1 -> UnitConverter1/1
  UnitConverter2/1 -> BitwiseOR/2
  SignalPack1/1 -> UnitConverter2/1
  UnitConverter3/1 -> SignalPack1/1
  convert_out/1 -> UnitConverter3/1
  Rr_IdcMin_toNidec/1 -> convert_out/1

== system halout/HAL_OUT/CAN3/FD3_VCU2_toNIDEC_0x154/Byte_4 ==
  Rr_IdcMin_toNidec : Inport
  BitwiseOR : simulink/Logic and Bit Operations/Bitwise Operator  logicop=OR  UseBitMask=off  BitMask=bin2dec('11011001')  BitMaskRealWorld=Stored Integer
  SignalPack : FVT_lib/hal/SignalPack  RightShiftCnt=0  BitMask=2^8-1  LeftShiftCnt=0
  UnitConverter : DataTypeConversion  OutDataTypeStr=uint8  RndMeth=Round
  UnitConverter1 : DataTypeConversion  OutDataTypeStr=uint16  RndMeth=Round
  convert_out : FVT_lib/hal/convert_out  gain=1  offset=-1022
  Byte_4 : Outport
  wires:
  BitwiseOR/1 -> Byte_4/1
  UnitConverter/1 -> BitwiseOR/1
  SignalPack/1 -> UnitConverter/1
  UnitConverter1/1 -> SignalPack/1
  convert_out/1 -> UnitConverter1/1
  Rr_IdcMin_toNidec/1 -> convert_out/1

== system halout/HAL_OUT/CAN3/FD3_VCU2_toNIDEC_0x154/Byte_5 ==
  Rr_TorqMax_toNidec : Inport
  BitwiseOR : simulink/Logic and Bit Operations/Bitwise Operator  logicop=OR  UseBitMask=off  BitMask=bin2dec('11011001')  BitMaskRealWorld=Stored Integer
  SignalPack : FVT_lib/hal/SignalPack  RightShiftCnt=4  BitMask=2^8-1  LeftShiftCnt=0
  UnitConverter : DataTypeConversion  OutDataTypeStr=uint8  RndMeth=Round
  UnitConverter1 : DataTypeConversion  OutDataTypeStr=uint16  RndMeth=Round
  Byte_5 : Outport
  wires:
  BitwiseOR/1 -> Byte_5/1
  UnitConverter/1 -> BitwiseOR/1
  SignalPack/1 -> UnitConverter/1
  UnitConverter1/1 -> SignalPack/1
  Rr_TorqMax_toNidec/1 -> UnitConverter1/1

== system halout/HAL_OUT/CAN3/FD3_VCU2_toNIDEC_0x154/Byte_6 ==
  Rr_TorqMax_toNidec : Inport
  Rr_TorqMin_toNidec : Inport  Port=2
  BitwiseOR : simulink/Logic and Bit Operations/Bitwise Operator  logicop=OR  UseBitMask=off  NumInputPorts=2  BitMask=bin2dec('11011001')  BitMaskRealWorld=Stored Integer
  SignalPack : FVT_lib/hal/SignalPack  RightShiftCnt=0  BitMask=2^4-1  LeftShiftCnt=4
  SignalPack1 : FVT_lib/hal/SignalPack  RightShiftCnt=8  BitMask=2^4-1  LeftShiftCnt=0
  UnitConverter : DataTypeConversion  OutDataTypeStr=uint8  RndMeth=Round
  UnitConverter1 : DataTypeConversion  OutDataTypeStr=uint16  RndMeth=Round
  UnitConverter2 : DataTypeConversion  OutDataTypeStr=uint8  RndMeth=Round
  UnitConverter3 : DataTypeConversion  OutDataTypeStr=uint16  RndMeth=Round
  convert_out : FVT_lib/hal/convert_out  gain=1  offset=-1022
  Byte_6 : Outport
  wires:
  BitwiseOR/1 -> Byte_6/1
  UnitConverter/1 -> BitwiseOR/1
  SignalPack/1 -> UnitConverter/1
  UnitConverter1/1 -> SignalPack/1
  Rr_TorqMax_toNidec/1 -> UnitConverter1/1
  UnitConverter2/1 -> BitwiseOR/2
  SignalPack1/1 -> UnitConverter2/1
  UnitConverter3/1 -> SignalPack1/1
  convert_out/1 -> UnitConverter3/1
  Rr_TorqMin_toNidec/1 -> convert_out/1

== system halout/HAL_OUT/CAN3/FD3_VCU2_toNIDEC_0x154/Byte_7 ==
  Rr_TorqMin_toNidec : Inport
  BitwiseOR : simulink/Logic and Bit Operations/Bitwise Operator  logicop=OR  UseBitMask=off  BitMask=bin2dec('11011001')  BitMaskRealWorld=Stored Integer
  SignalPack : FVT_lib/hal/SignalPack  RightShiftCnt=0  BitMask=2^8-1  LeftShiftCnt=0
  UnitConverter : DataTypeConversion  OutDataTypeStr=uint8  RndMeth=Round
  UnitConverter1 : DataTypeConversion  OutDataTypeStr=uint16  RndMeth=Round
  convert_out : FVT_lib/hal/convert_out  gain=1  offset=-1022
  Byte_7 : Outport
  wires:
  BitwiseOR/1 -> Byte_7/1
  UnitConverter/1 -> BitwiseOR/1
  SignalPack/1 -> UnitConverter/1
  UnitConverter1/1 -> SignalPack/1
  convert_out/1 -> UnitConverter1/1
  Rr_TorqMin_toNidec/1 -> convert_out/1

== system halout/HAL_OUT/CAN3/FD3_VCU2_toNIDEC_0x154/Byte_8 ==
  Rr_UdcMax_toNidec : Inport
  BitwiseOR : simulink/Logic and Bit Operations/Bitwise Operator  logicop=OR  UseBitMask=off  BitMask=bin2dec('11011001')  BitMaskRealWorld=Stored Integer
  SignalPack : FVT_lib/hal/SignalPack  RightShiftCnt=4  BitMask=2^8-1  LeftShiftCnt=0
  UnitConverter : DataTypeConversion  OutDataTypeStr=uint8  RndMeth=Round
  UnitConverter1 : DataTypeConversion  OutDataTypeStr=uint16  RndMeth=Round
  Byte_8 : Outport
  wires:
  BitwiseOR/1 -> Byte_8/1
  UnitConverter/1 -> BitwiseOR/1
  SignalPack/1 -> UnitConverter/1
  UnitConverter1/1 -> SignalPack/1
  Rr_UdcMax_toNidec/1 -> UnitConverter1/1

== system halout/HAL_OUT/CAN3/FD3_VCU2_toNIDEC_0x154/Byte_9 ==
  Rr_UdcMax_toNidec : Inport
  Rr_UdcMin_toNidec : Inport  Port=2
  BitwiseOR : simulink/Logic and Bit Operations/Bitwise Operator  logicop=OR  UseBitMask=off  NumInputPorts=2  BitMask=bin2dec('11011001')  BitMaskRealWorld=Stored Integer
  SignalPack : FVT_lib/hal/SignalPack  RightShiftCnt=0  BitMask=2^4-1  LeftShiftCnt=4
  SignalPack1 : FVT_lib/hal/SignalPack  RightShiftCnt=8  BitMask=2^4-1  LeftShiftCnt=0
  UnitConverter : DataTypeConversion  OutDataTypeStr=uint8  RndMeth=Round
  UnitConverter1 : DataTypeConversion  OutDataTypeStr=uint16  RndMeth=Round
  UnitConverter2 : DataTypeConversion  OutDataTypeStr=uint8  RndMeth=Round
  UnitConverter3 : DataTypeConversion  OutDataTypeStr=uint16  RndMeth=Round
  Byte_9 : Outport
  wires:
  BitwiseOR/1 -> Byte_9/1
  UnitConverter/1 -> BitwiseOR/1
  SignalPack/1 -> UnitConverter/1
  UnitConverter1/1 -> SignalPack/1
  Rr_UdcMax_toNidec/1 -> UnitConverter1/1
  UnitConverter2/1 -> BitwiseOR/2
  SignalPack1/1 -> UnitConverter2/1
  UnitConverter3/1 -> SignalPack1/1
  Rr_UdcMin_toNidec/1 -> UnitConverter3/1

== system halout/HAL_OUT/CAN3/FD3_VCU2_toNIDEC_0x154/CRC8_IfAction_Tx ==
  CAN_E2E_flg : Inport
  DataID1 : Inport  Port=2
  DataID2 : Inport  Port=3
  RawData : Inport  Port=4
  Data Type Conversion : DataTypeConversion  OutDataTypeStr=uint8
  If : If
  If Action Subsystem : Subsystem  TreatAsAtomicUnit=on
  If Action Subsystem1 : Subsystem  TreatAsAtomicUnit=on
  Merge : Merge
  CRC8 : Outport
  wires:
  If/2 -> If Action Subsystem/Action
  If/1 -> If Action Subsystem1/Action
  CAN_E2E_flg/1 -> [CAN_E2E_flg]
  DataID1/1 -> [DataID1]
  DataID2/1 -> [DataID2]
  RawData/1 -> [RawData]
  [CAN_E2E_flg] -> Data Type Conversion/1
  [DataID1] -> If Action Subsystem1/1(CAN_E2E_ID1)
  [DataID2] -> If Action Subsystem1/2(CAN_E2E_ID2)
  [RawData] -> If Action Subsystem1/3(Byte1)
  [RawData] -> If Action Subsystem/1(Byte1)
  If Action Subsystem1/1(CRC8_E2EResult) -> Merge/1
  If Action Subsystem/1(CRC8_Result) -> Merge/2
  Merge/1 -> CRC8/1
  Data Type Conversion/1 -> If/1

== system halout/HAL_OUT/CAN3/FD3_VCU2_toNIDEC_0x154/CSVCU2CAN1toNidec ==
  CSVCU2CAN1toNidec : Inport
  Data Type Conversion : DataTypeConversion  OutDataTypeStr=uint8  RndMeth=Round
  CAN3_CS_VCU2_CAN1_toNidec : Outport
  wires:
  Data Type Conversion/1 -> CAN3_CS_VCU2_CAN1_toNidec/1
  CSVCU2CAN1toNidec/1 -> Data Type Conversion/1

== system halout/HAL_OUT/CAN3/FD3_VCU2_toNIDEC_0x154/FrIdcMaxtoNidec ==
  FrIdcMaxtoNidec : Inport
  Data Type Conversion : DataTypeConversion  OutDataTypeStr=uint16  RndMeth=Round
  CAN3_Fr_IdcMax_toNidec : Outport
  wires:
  Data Type Conversion/1 -> CAN3_Fr_IdcMax_toNidec/1
  FrIdcMaxtoNidec/1 -> Data Type Conversion/1

== system halout/HAL_OUT/CAN3/FD3_VCU2_toNIDEC_0x154/FrIdcMintoNidec ==
  FrIdcMintoNidec : Inport
  Data Type Conversion : DataTypeConversion  OutDataTypeStr=uint16  RndMeth=Round
  convert_out : FVT_lib/hal/convert_out  gain=1  offset=-1022
  CAN3_Fr_IdcMin_toNidec : Outport
  wires:
  Data Type Conversion/1 -> CAN3_Fr_IdcMin_toNidec/1
  convert_out/1 -> Data Type Conversion/1
  FrIdcMintoNidec/1 -> convert_out/1

== system halout/HAL_OUT/CAN3/FD3_VCU2_toNIDEC_0x154/FrTMTqReqtoNidec ==
  FrTMTqReqtoNidec : Inport
  Data Type Conversion : DataTypeConversion  OutDataTypeStr=uint16  RndMeth=Round
  convert_out : FVT_lib/hal/convert_out  gain=1  offset=-530
  CAN3_Fr_TMTqReq_toNidec : Outport
  wires:
  Data Type Conversion/1 -> CAN3_Fr_TMTqReq_toNidec/1
  convert_out/1 -> Data Type Conversion/1
  FrTMTqReqtoNidec/1 -> convert_out/1

== system halout/HAL_OUT/CAN3/FD3_VCU2_toNIDEC_0x154/FrTorqMaxtoNidec ==
  FrTorqMaxtoNidec : Inport
  Data Type Conversion : DataTypeConversion  OutDataTypeStr=uint16  RndMeth=Round
  CAN3_Fr_TorqMax_toNidec : Outport
  wires:
  Data Type Conversion/1 -> CAN3_Fr_TorqMax_toNidec/1
  FrTorqMaxtoNidec/1 -> Data Type Conversion/1
